simulink model "SubsystemTest3"  (R2020b)
settings: Solver=FixedStepAuto  StartTime=0.0  StopTime=72  FixedStep=0.1  RelTol=1e-3
settings Model: Creator=jim  LastModifiedBy=jimd

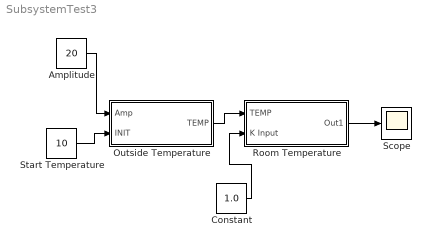
== system SubsystemTest3 ==
  Amplitude : Constant  Value=20
  Constant : Constant  Value=1.0
  Outside Temperature : Subsystem
  Room Temperature : Subsystem
  Scope : Scope
  Start Temperature : Constant  Value=10
  wires:
  Amplitude/1 -> Outside Temperature/1(Amp)
  Start Temperature/1 -> Outside Temperature/2(INIT)
  Outside Temperature/1(TEMP) -> Room Temperature/1(TEMP)
  Room Temperature/1(Out1) -> Scope/1
  Constant/1 -> Room Temperature/2(K Input)

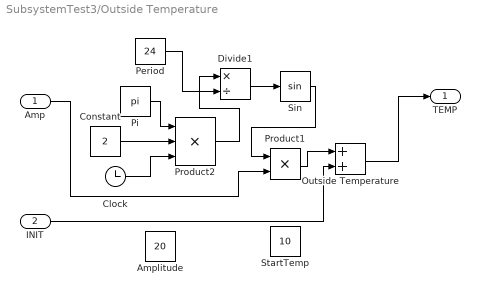
== system SubsystemTest3/Outside Temperature ==
  Amp : Inport
  INIT : Inport  Port=2
  Amplitude : Constant  Value=20
  Clock : Clock
  Constant : Constant  Value=2
  Divide1 : Product  Inputs=*/
  Outside Temperature : Sum
  Period : Constant  Value=24
  Pi : Constant  Value=pi  OutDataTypeStr=Inherit: Inherit via back propagation
  Product1 : Product
  Product2 : Product  Inputs=3
  Sin : Trigonometry
  StartTemp : Constant  Value=10
  TEMP : Outport
  wires:
  Divide1/1 -> Sin/1
  Product2/1 -> Divide1/1
  Constant/1 -> Product2/2
  Sin/1 -> Product1/1
  Pi/1 -> Product2/1
  Clock/1 -> Product2/3
  Period/1 -> Divide1/2
  Product1/1 -> Outside Temperature/1
  Outside Temperature/1 -> TEMP/1
  Amp/1 -> Product1/2
  INIT/1 -> Outside Temperature/2

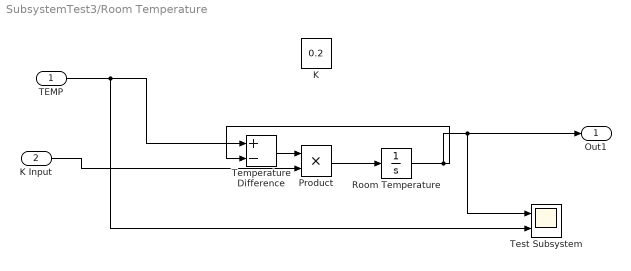
== system SubsystemTest3/Room Temperature ==
  TEMP : Inport
  K Input : Inport  Port=2
  K : Constant  Value=0.2
  Product : Product
  Room Temperature : Integrator  InitialCondition=10
  Temperature Difference : Sum  Inputs=+-
  Test Subsystem : Scope  NumInputPorts=2
  Out1 : Outport
  wires:
  Product/1 -> Room Temperature/1
  Temperature Difference/1 -> Product/1
  Room Temperature/1 -> Test Subsystem/1, Out1/1, Temperature Difference/2
  TEMP/1 -> Test Subsystem/2, Temperature Difference/1
  K Input/1 -> Product/2
